simulink model "CryoDetXray"  (R2016b)
settings: Solver=ode45  StartTime=0.0  StopTime=10e-5  MaxStep=Tclk/4  RelTol=1e-3
values from neighbouring files (symbols this model uses):
  Fclk = Fadc    (= 307200000)    [setupCryoFPGAxray.m]
  Tclk = 1/Fclk    (= 3.25520833333e-09)    [setupCryoFPGAxray.m]
undefined symbols (not defined in the file or in its folder): AXI4, Lite, lpf, Naxi, xlipgetpartsetting
libraries: xbsIndex_r4 x1091, CryoDetLib x68, simulink x4, hdlsllib x1
(part 7 of 8)

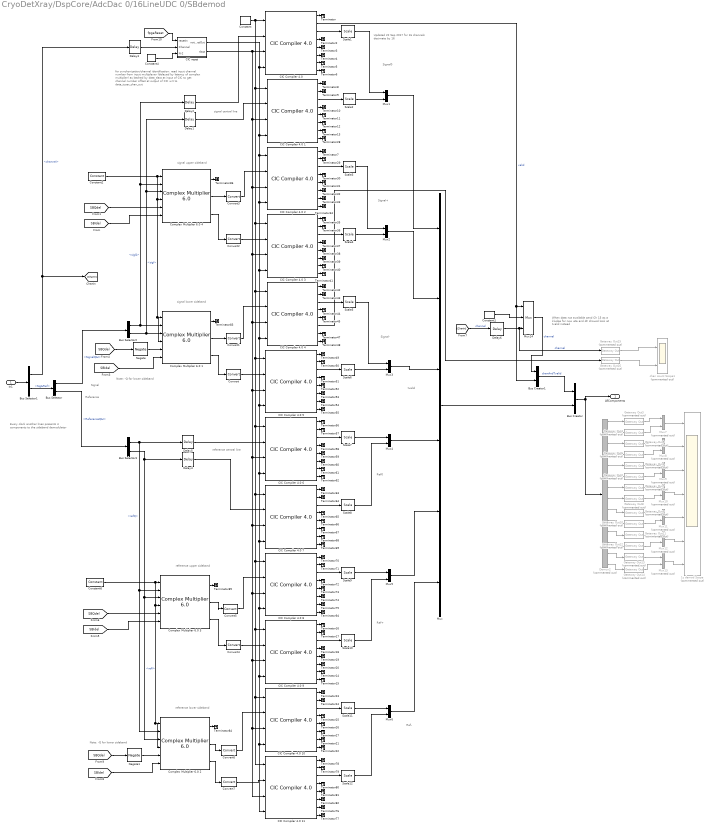
== system CryoDetXray/DspCore/AdcDac 0/16LineUDC 0/SBdemod ==
  note: Updated 22 Sep 2017 for 16 channels
      | decimate by 16
  note: When data not available send Ch 15 as
      | a kludge for now
      | eta and dF shouod look at tvalid instead
  note: tvalid
  note: Ref-
  note: Ref+
  note: Ref0
  note: Signal-
  note: Signal+
  note: Signal0
  note: for synchonization/channel identification:
      | read input channel number  from input multiplexer (delayed by latency of complex multiplier)
      | as latched by data_tlast at input of CIC to get channel number offset at output of CIC wrt to data_tuser_chan_out
  note: Note: -Q for lower sideband
  note: Every clock another lines presents 4 components to the sideband demodulator
  note: signal
      | central line
  note: signal
      | upper sideband
  note: signal
      | lower sideband
  note: Signal
  note: Reference
  note: reference
      | central line
  note: reference
      | upper sideband
  note: reference
      | lower sideband
  note: Note: -Q for lower sideband
  In1 : Inport
  1c demod Scope : Scope  Commented=on  NumInputPorts=7
  Bus Creator : BusCreator  Inputs=2
  Bus Creator1 : BusCreator  Inputs=2
  Bus Selector : BusSelector  OutputSignals=SignalQ&I,ReferenceQ&I
  Bus Selector1 : BusSelector  OutputSignals=channel,Sig&Ref
  Bus Selector2 : BusSelector  OutputSignals=sigQ,sigI
  Bus Selector3 : BusSelector  OutputSignals=refQ,refI
  CIC Compiler 4.0 {,1..11} (12 alike) : xbsIndex_r4/CIC Compiler 4.0   filter_type=Decimation  number_of_stages=3  differential_delay=1  number_of_channels=16  sample_rate_changes=Fixed  fixed_or_initial_rate=16  minimum_rate=16  maximum_rate=16  ratespecification=Sample_Period  sampleperiod=1  hardwareoversamplingrate=1  quantization=Truncation  output_data_width=24  use_xtreme_dsp_slice=off  use_streaming_interface=off  has_aclken=off  has_aresetn=on  has_dout_tready=off  trim_axipin_name=on  gui_behaviour=Sysgen_GUI  input_data_width=18  ip_name=CIC Compiler  ip_version=4.0  dsptool_ready=true  wrapper_available=true  port_translation_map={ 'aclken' => 'en', 'aresetn' => 'rst' }  ipcore_xco_need_fpga_part=true  ipcore_verbose=false  block_type=cic_compiler_v4_0
  CIC reset : Subsystem
  Complex Multiplier 6.0 {1..4} (4 alike) : xbsIndex_r4/Complex Multiplier 6.0   hasatlast=off  hasatuser=off  atuserwidth=1  hasbtlast=off  hasbtuser=off  btuserwidth=1  multtype=Use_Mults  optimizegoal=Resources  flowcontrol=NonBlocking  outputwidth=23  roundmode=Truncate  hasctrltlast=off  hasctrltuser=off  ctrltuserwidth=1  outtlastbehv=Null  latencyconfig=Manual  minimumlatency=6  aclken=off  aresetn=off  trim_axipin_name=on  simulation_type=hybrid_sim  simulation_model=sysgen:cmpy_v6_0  data_path_portlist={ 's_axis_a_tdata_real', 's_axis_a_tdata_imag', 's_axis_b_tdata_real', 's_axis_b_tdata_imag', 's_axis_ctrl_tdata_rounding_bit', 'm_axis_dout_tdata_real', 'm_axis_dout_tdata_imag' }  aportwidth=63  bportwidth=63  ip_name=Complex Multiplier  ip_version=6.0  dsptool_ready=true  ipcore_usecache=true  ipcore_useipmodelcache=true  ipcore_verbose=false  ipcore_latency_parameter='minimumlatency'  wrapper_available=true  port_translation_map={ 'aclken' => 'en', 'aresetn' => 'rst'}  block_type=cmpy_v6_0
  Constant : xbsIndex_r4/Constant  const=1.0  gui_display_data_type=Boolean  arith_type=Boolean  n_bits=16  bin_pt=14  preci_type=Single  exp_width=8  frac_width=24  explicit_period=off  period=1  equ=P=C  opselect=C  inp2=PCIN>>17  opr=+  inp1=P  carry=CIN  dbl_ovrd=off  block_type=constant
  Constant1 : xbsIndex_r4/Constant  const=15  gui_display_data_type=Fixed-point  arith_type=Unsigned  n_bits=4  bin_pt=0  preci_type=Single  exp_width=8  frac_width=24  explicit_period=off  period=1  equ=P=C  opselect=C  inp2=PCIN>>17  opr=+  inp1=P  carry=CIN  dbl_ovrd=off  block_type=constant
  Constant2 : xbsIndex_r4/Constant  const=1.0  gui_display_data_type=Boolean  arith_type=Boolean  n_bits=16  bin_pt=14  preci_type=Single  exp_width=8  frac_width=24  explicit_period=off  period=1  equ=P=C  opselect=C  inp2=PCIN>>17  opr=+  inp1=P  carry=CIN  dbl_ovrd=off  block_type=constant
  Constant4 : xbsIndex_r4/Constant  const=14  gui_display_data_type=Fixed-point  arith_type=Unsigned  n_bits=4  bin_pt=0  preci_type=Single  exp_width=8  frac_width=24  explicit_period=off  period=1  equ=P=C  opselect=C  inp2=PCIN>>17  opr=+  inp1=P  carry=CIN  dbl_ovrd=off  block_type=constant
  Constant6 : xbsIndex_r4/Constant  const=1.0  gui_display_data_type=Boolean  arith_type=Boolean  n_bits=16  bin_pt=14  preci_type=Single  exp_width=8  frac_width=24  explicit_period=off  period=1  equ=P=C  opselect=C  inp2=PCIN>>17  opr=+  inp1=P  carry=CIN  dbl_ovrd=off  block_type=constant
  Convert{,1..7} (8 alike) : xbsIndex_r4/Convert  gui_display_data_type=Fixed-point  arith_type="Signed  (2's comp)"  n_bits=20  bin_pt=16  float_type=Single  exp_bits=8  fraction_bits=24  quantization="Round  (unbiased: +/- Inf)"  overflow=Saturate  en=off  latency=0  pipeline=off  dbl_ovrd=off  block_type=convert
  Delay{1..2,4..5} (4 alike) : xbsIndex_r4/Delay  rst=off  infoeditControl=Selection of Reset will increase slice count due to use of real FFs and instead of SRLs  en=off  latency=6  reg_retiming=off  dbl_ovrd=off  block_type=delay
  Delay3 : xbsIndex_r4/Delay  rst=off  infoeditControl=Selection of Reset will increase slice count due to use of real FFs and instead of SRLs  en=off  latency=6  reg_retiming=on  dbl_ovrd=off  block_type=delay
  Delay6 : xbsIndex_r4/Delay  rst=off  infoeditControl=Selection of Reset will increase slice count due to use of real FFs and instead of SRLs  en=off  latency=4  reg_retiming=off  dbl_ovrd=off  block_type=delay
  Demux2 : Demux  Commented=on  Outputs=14
  Gateway Out{1..16} (16 alike) : xbsIndex_r4/Gateway Out  Commented=on  inherit_from_input=off  hdl_port=off  rows=1  columns=1  UseAsDAC=off  DACChannel='1'  interface=None  automatic_assignment=on  address_offset=hex2dec('00')  intf_name=''  intf_description=''  timing_constraint=None  locs_specified=off  LOCs={}  io_standard={}  block_type=gatewayout
  Mux : Mux  Inputs=6
  Mux{1..6} (6 alike) : Mux  Inputs=2
  Mux{7..13} (7 alike) : Mux  Commented=on  Inputs=2
  Mux14 : xbsIndex_r4/Mux  inputs=2  en=off  latency=0  precision=Full  arith_type=Unsigned  n_bits=16  bin_pt=14  quantization=Truncate  overflow=Wrap  dbl_ovrd=off  block_type=mux
  Negate : xbsIndex_r4/Negate  precision=User Defined  arith_type="Signed  (2's comp)"  n_bits=16  bin_pt=14  quantization=Truncate  overflow=Wrap  en=off  latency=0  dbl_ovrd=off  block_type=negate
  Negate1 : xbsIndex_r4/Negate  precision=User Defined  arith_type="Signed  (2's comp)"  n_bits=16  bin_pt=14  quantization=Truncate  overflow=Wrap  en=off  latency=0  dbl_ovrd=off  block_type=negate
  Scale{1..12} (12 alike) : xbsIndex_r4/Scale  scale_factor=-12  dbl_ovrd=off  block_type=scale
  Terminator{,2..45,47..86,94} (86 alike) : Terminator
  chan count Scope1 : Scope  Commented=on  NumInputPorts=2
  AllComponents : Outport
  wires:
  "CIC Compiler 4.0 "/3 -> Scale1/1
  Bus Selector/1 -> Bus Selector2/1  "<SignalQ&I>"
  Bus Selector2/1 -> Delay2/1, Complex Multiplier 6.0 4/2, Complex Multiplier 6.0 1/2  "<sigQ>"
  Bus Selector2/2 -> Complex Multiplier 6.0 4/3, Delay1/1, Complex Multiplier 6.0 1/3  "<sigI>"
  Bus Selector/2 -> Bus Selector3/1  "<ReferenceQ&I>"
  [SBIdel] -> Complex Multiplier 6.0 4/6
  [SBQdel] -> Complex Multiplier 6.0 4/5
  CIC reset/2(tlast) -> CIC Compiler 4.0 1/3, CIC Compiler 4.0 2/3, CIC Compiler 4.0 3/3, CIC Compiler 4.0 4/3, CIC Compiler 4.0 5/3, CIC Compiler 4.0 6/3, CIC Compiler 4.0 7/3, CIC Compiler 4.0 8/3, CIC Compiler 4.0 9/3, CIC Compiler 4.0 11/3, CIC Compiler 4.0 10/3, "CIC Compiler 4.0 "/3
  CIC reset/1(notResetOut) -> CIC Compiler 4.0 1/4, CIC Compiler 4.0 2/1, CIC Compiler 4.0 2/4, CIC Compiler 4.0 3/4, CIC Compiler 4.0 4/4, CIC Compiler 4.0 5/4, CIC Compiler 4.0 6/4, CIC Compiler 4.0 7/4, CIC Compiler 4.0 8/4, CIC Compiler 4.0 9/4, CIC Compiler 4.0 11/4, CIC Compiler 4.0 10/4, "CIC Compiler 4.0 "/4
  In1/1 -> Bus Selector1/1
  Bus Selector1/2 -> Bus Selector/1  "<Sig&Ref>"
  Delay1/1 -> CIC Compiler 4.0 1/2
  Delay2/1 -> "CIC Compiler 4.0 "/2
  Complex Multiplier 6.0 4/2 -> Convert3/1
  Complex Multiplier 6.0 4/3 -> Convert2/1
  Complex Multiplier 6.0 1/2 -> Convert1/1
  Complex Multiplier 6.0 1/3 -> Convert/1
  Constant2/1 -> Complex Multiplier 6.0 4/4, Complex Multiplier 6.0 1/4, Complex Multiplier 6.0 1/1, Complex Multiplier 6.0 4/1
  Bus Selector3/1 -> Complex Multiplier 6.0 2/2, Complex Multiplier 6.0 3/2, Delay5/1  "<refQ>"
  Bus Selector3/2 -> Complex Multiplier 6.0 2/3, Complex Multiplier 6.0 3/3, Delay4/1  "<refI>"
  [SBIdel] -> Complex Multiplier 6.0 3/6
  [SBQdel] -> Complex Multiplier 6.0 3/5
  Constant/1 -> "CIC Compiler 4.0 "/1, CIC Compiler 4.0 1/1, CIC Compiler 4.0 3/1, CIC Compiler 4.0 4/1, CIC Compiler 4.0 5/1, CIC Compiler 4.0 6/1, CIC Compiler 4.0 7/1, CIC Compiler 4.0 8/1, CIC Compiler 4.0 9/1, CIC Compiler 4.0 11/1, CIC Compiler 4.0 10/1
  Delay4/1 -> CIC Compiler 4.0 7/2
  Delay5/1 -> CIC Compiler 4.0 6/2
  Complex Multiplier 6.0 3/2 -> Convert5/1
  Complex Multiplier 6.0 3/3 -> Convert4/1
  Complex Multiplier 6.0 2/2 -> Convert6/1
  Complex Multiplier 6.0 2/3 -> Convert7/1
  Constant6/1 -> Complex Multiplier 6.0 3/4, Complex Multiplier 6.0 2/4, Complex Multiplier 6.0 2/1, Complex Multiplier 6.0 3/1
  Bus Selector1/1 -> Delay3/1, [ChanIn]  "<channel>"
  Delay3/1 -> CIC reset/2(Channel)
  Scale1/1 -> Mux1/1
  Scale6/1 -> Mux3/2
  Scale7/1 -> Mux4/1
  Scale8/1 -> Mux4/2
  Scale9/1 -> Mux5/1
  Scale10/1 -> Mux5/2
  Scale11/1 -> Mux6/1
  Scale12/1 -> Mux6/2
  Mux6/1 -> Mux/6
  Mux5/1 -> Mux/5
  Mux4/1 -> Mux/4
  Mux3/1 -> Mux/3
  Mux2/1 -> Mux/2
  Mux1/1 -> Mux/1
  Mux/1 -> Bus Creator/2
  [ChanIn] -> Delay6/1  "channel"
  Bus Creator1/1 -> Bus Creator/1  "chanAndTvalid"
  Convert/1 -> CIC Compiler 4.0 5/2
  Convert1/1 -> CIC Compiler 4.0 4/2
  Convert2/1 -> CIC Compiler 4.0 3/2
  Convert3/1 -> CIC Compiler 4.0 2/2
  Convert4/1 -> CIC Compiler 4.0 9/2
  Convert5/1 -> CIC Compiler 4.0 8/2
  Convert7/1 -> CIC Compiler 4.0 11/2
  Convert6/1 -> CIC Compiler 4.0 10/2
  Bus Creator/1 -> AllComponents/1, Demux2/1
  Demux2/1 -> Gateway Out3/1
  Demux2/2 -> Gateway Out4/1
  Demux2/3 -> Gateway Out5/1
  Demux2/4 -> Gateway Out6/1
  Gateway Out6/1 -> Mux8/2
  Gateway Out5/1 -> Mux8/1
  Gateway Out4/1 -> Mux7/2
  Gateway Out3/1 -> Mux7/1
  Mux7/1 -> 1c demod Scope/1
  Mux8/1 -> 1c demod Scope/2
  Demux2/14 -> Gateway Out14/1
  Demux2/13 -> Gateway Out13/1
  Gateway Out13/1 -> Mux13/1
  Gateway Out14/1 -> Mux13/2
  Mux13/1 -> 1c demod Scope/7
  Demux2/12 -> Gateway Out12/1
  Demux2/11 -> Gateway Out11/1
  Gateway Out11/1 -> Mux12/1
  Gateway Out12/1 -> Mux12/2
  Mux12/1 -> 1c demod Scope/6
  Demux2/10 -> Gateway Out10/1
  Demux2/9 -> Gateway Out9/1
  Gateway Out9/1 -> Mux11/1
  Gateway Out10/1 -> Mux11/2
  Mux11/1 -> 1c demod Scope/5
  Demux2/8 -> Gateway Out8/1
  Gateway Out8/1 -> Mux10/2
  Mux10/1 -> 1c demod Scope/4
  Gateway Out7/1 -> Mux10/1
  Demux2/7 -> Gateway Out7/1
  Demux2/6 -> Gateway Out2/1
  Gateway Out2/1 -> Mux9/2
  Gateway Out1/1 -> Mux9/1
  Demux2/5 -> Gateway Out1/1
  Mux9/1 -> 1c demod Scope/3
  Constant4/1 -> CIC reset/3(N-2)
  [fpgaReset] -> CIC reset/1(resetIn)
  Delay6/1 -> Gateway Out15/1, Mux14/3  "channel"
  Constant1/1 -> Mux14/2
  Mux14/1 -> Bus Creator1/1  "channel"
  [SBIdel] -> Complex Multiplier 6.0 1/6
  Negate/1 -> Complex Multiplier 6.0 1/5
  [SBQdel] -> Negate/1
  [SBIdel] -> Complex Multiplier 6.0 2/6
  [SBQdel] -> Negate1/1
  Negate1/1 -> Complex Multiplier 6.0 2/5
  "CIC Compiler 4.0 "/1 -> Terminator/1
  "CIC Compiler 4.0 "/2 -> Mux14/1, Bus Creator1/2  "valid"
  "CIC Compiler 4.0 "/4 -> Terminator2/1
  "CIC Compiler 4.0 "/5 -> Terminator3/1
  "CIC Compiler 4.0 "/6 -> Terminator4/1
  "CIC Compiler 4.0 "/7 -> Terminator5/1
  "CIC Compiler 4.0 "/8 -> Terminator6/1
  Complex Multiplier 6.0 1/1 -> Terminator83/1
  Complex Multiplier 6.0 2/1 -> Terminator84/1
  Complex Multiplier 6.0 3/1 -> Terminator85/1
  Complex Multiplier 6.0 4/1 -> Terminator86/1
  CIC Compiler 4.0 1/3 -> Scale2/1
  CIC Compiler 4.0 1/1 -> Terminator8/1
  CIC Compiler 4.0 1/2 -> Terminator9/1
  CIC Compiler 4.0 1/4 -> Terminator10/1
  CIC Compiler 4.0 1/5 -> Terminator11/1
  CIC Compiler 4.0 1/6 -> Terminator12/1
  CIC Compiler 4.0 1/7 -> Terminator13/1
  CIC Compiler 4.0 1/8 -> Terminator28/1
  CIC Compiler 4.0 2/3 -> Scale3/1
  CIC Compiler 4.0 2/1 -> Terminator7/1
  CIC Compiler 4.0 2/2 -> Terminator29/1
  CIC Compiler 4.0 2/4 -> Terminator30/1
  CIC Compiler 4.0 2/5 -> Terminator31/1
  CIC Compiler 4.0 2/6 -> Terminator32/1
  CIC Compiler 4.0 2/7 -> Terminator33/1
  CIC Compiler 4.0 2/8 -> Terminator34/1
  CIC Compiler 4.0 3/3 -> Scale4/1
  CIC Compiler 4.0 3/1 -> Terminator35/1
  CIC Compiler 4.0 3/2 -> Terminator36/1
  CIC Compiler 4.0 3/4 -> Terminator37/1
  CIC Compiler 4.0 3/5 -> Terminator38/1
  CIC Compiler 4.0 3/6 -> Terminator39/1
  CIC Compiler 4.0 3/7 -> Terminator40/1
  CIC Compiler 4.0 3/8 -> Terminator41/1
  CIC Compiler 4.0 4/3 -> Scale5/1
  CIC Compiler 4.0 4/1 -> Terminator42/1
  CIC Compiler 4.0 4/2 -> Terminator43/1
  CIC Compiler 4.0 4/4 -> Terminator44/1
  CIC Compiler 4.0 4/5 -> Terminator45/1
  CIC Compiler 4.0 4/7 -> Terminator47/1
  CIC Compiler 4.0 4/8 -> Terminator48/1
  Scale2/1 -> Mux1/2
  Scale3/1 -> Mux2/1
  Scale4/1 -> Mux2/2
  Scale5/1 -> Mux3/1
  CIC Compiler 4.0 5/3 -> Scale6/1
  CIC Compiler 4.0 5/1 -> Terminator49/1
  CIC Compiler 4.0 5/2 -> Terminator50/1
  CIC Compiler 4.0 5/4 -> Terminator51/1
  CIC Compiler 4.0 5/5 -> Terminator52/1
  CIC Compiler 4.0 5/6 -> Terminator53/1
  CIC Compiler 4.0 5/7 -> Terminator54/1
  CIC Compiler 4.0 5/8 -> Terminator55/1
  CIC Compiler 4.0 6/3 -> Scale7/1
  CIC Compiler 4.0 6/1 -> Terminator56/1
  CIC Compiler 4.0 6/2 -> Terminator57/1
  CIC Compiler 4.0 6/4 -> Terminator58/1
  CIC Compiler 4.0 6/5 -> Terminator59/1
  CIC Compiler 4.0 6/6 -> Terminator60/1
  CIC Compiler 4.0 6/7 -> Terminator61/1
  CIC Compiler 4.0 6/8 -> Terminator62/1
  CIC Compiler 4.0 7/3 -> Scale8/1
  CIC Compiler 4.0 7/1 -> Terminator63/1
  CIC Compiler 4.0 7/2 -> Terminator64/1
  CIC Compiler 4.0 7/4 -> Terminator65/1
  CIC Compiler 4.0 7/5 -> Terminator66/1
  CIC Compiler 4.0 7/6 -> Terminator67/1
  CIC Compiler 4.0 7/7 -> Terminator68/1
  CIC Compiler 4.0 7/8 -> Terminator69/1
  CIC Compiler 4.0 8/3 -> Scale9/1
  CIC Compiler 4.0 8/1 -> Terminator70/1
  CIC Compiler 4.0 8/2 -> Terminator71/1
  CIC Compiler 4.0 8/4 -> Terminator72/1
  CIC Compiler 4.0 8/5 -> Terminator73/1
  CIC Compiler 4.0 8/6 -> Terminator74/1
  CIC Compiler 4.0 8/7 -> Terminator75/1
  CIC Compiler 4.0 8/8 -> Terminator94/1
  CIC Compiler 4.0 9/3 -> Scale10/1
  CIC Compiler 4.0 9/1 -> Terminator16/1
  CIC Compiler 4.0 9/2 -> Terminator17/1
  CIC Compiler 4.0 9/4 -> Terminator18/1
  CIC Compiler 4.0 9/5 -> Terminator19/1
  CIC Compiler 4.0 9/6 -> Terminator20/1
  CIC Compiler 4.0 9/7 -> Terminator14/1
  CIC Compiler 4.0 9/8 -> Terminator15/1
  CIC Compiler 4.0 10/3 -> Scale11/1
  CIC Compiler 4.0 10/1 -> Terminator23/1
  CIC Compiler 4.0 10/2 -> Terminator24/1
  CIC Compiler 4.0 10/4 -> Terminator25/1
  CIC Compiler 4.0 10/5 -> Terminator26/1
  CIC Compiler 4.0 10/6 -> Terminator27/1
  CIC Compiler 4.0 10/7 -> Terminator21/1
  CIC Compiler 4.0 10/8 -> Terminator22/1
  CIC Compiler 4.0 11/3 -> Scale12/1
  CIC Compiler 4.0 11/1 -> Terminator78/1
  CIC Compiler 4.0 11/2 -> Terminator79/1
  CIC Compiler 4.0 11/4 -> Terminator80/1
  CIC Compiler 4.0 11/5 -> Terminator81/1
  CIC Compiler 4.0 11/6 -> Terminator82/1
  CIC Compiler 4.0 11/7 -> Terminator76/1
  CIC Compiler 4.0 11/8 -> Terminator77/1
  CIC Compiler 4.0 4/6 -> Gateway Out16/1
  Gateway Out15/1 -> chan count Scope1/1
  Gateway Out16/1 -> chan count Scope1/2

== system CryoDetXray/DspCore/AdcDac 0/16LineUDC 0/debug Scope ==
  note: Debug Demodulation
  demod : Inport
  freq : Inport  Port=2
  Complex to Magnitude-Angle : ComplexToMagnitudeAngle  Output=Magnitude
  Demux1 : Demux
  Gain : Gain  Gain=Fclk
  Gateway Out{1,3..6} (5 alike) : xbsIndex_r4/Gateway Out  inherit_from_input=off  hdl_port=off  rows=1  columns=1  UseAsDAC=off  DACChannel='1'  interface=None  automatic_assignment=on  address_offset=hex2dec('00')  intf_name=''  intf_description=''  timing_constraint=None  locs_specified=off  LOCs={}  io_standard={}  block_type=gatewayout
  Mux4 : Mux  Inputs=3
  Mux5 : Mux  Inputs=2
  Real-Imag to Complex : RealImagToComplex
  block downconverter Scope : Scope  NumInputPorts=3
  tag scope: FreqCh0=global
  wires:
  Gain/1 -> [FreqCh0], block downconverter Scope/3
  Gateway Out1/1 -> Gain/1
  freq/1 -> Gateway Out1/1
  Real-Imag to Complex/1 -> Complex to Magnitude-Angle/1
  Complex to Magnitude-Angle/1 -> Mux4/3
  Mux5/1 -> block downconverter Scope/2
  Mux4/1 -> block downconverter Scope/1
  Gateway Out3/1 -> Real-Imag to Complex/2, Mux4/1
  Gateway Out4/1 -> Real-Imag to Complex/1, Mux4/2
  Gateway Out5/1 -> Mux5/1
  Gateway Out6/1 -> Mux5/2
  Demux1/4 -> Gateway Out6/1
  Demux1/3 -> Gateway Out5/1
  Demux1/2 -> Gateway Out4/1
  Demux1/1 -> Gateway Out3/1
  demod/1 -> Demux1/1

== system CryoDetXray/DspCore/AdcDac 0/16ch LBW LPF/CIC reset ==
  note: where N is number of channels in CIC filter
  note: reset latched resetIn
  note: latch resetIn
  note: CIC reset
      |
      | Synchronizes a CIC compiler 4.0 multi-channel CIC filter
      | to input channels
      |
      | Generates:
      | 1	notResetOut to CIC aresetn
      | 2	tlast to CIC tlast input
      |
      | Inputs:
      | 1	reset in
      | 2	Channel number (0-N) which may go to sel input of mux generating the input data stream
      | 3	N-2 which tells this module how deep is the multiplexing (e.g. N-2 = 10 for a 12 channel CIC filter (sorry))
      |
      | Guarantees:
      | 1	reset out is at least 2 clocks long
      | 2	end of reset occurs 2 clocks before channel 0
      | 3	tlast comes with channel N-1
      |
      | Assumes:
      | CIC oversampling set to "Sample period" = 1
      | No "streaming interface"
  resetIn : Inport
  Channel : Inport  Port=2
  N-2 : Inport  Port=3
  Constant : xbsIndex_r4/Constant  const=0  gui_display_data_type=Boolean  arith_type=Boolean  n_bits=16  bin_pt=14  preci_type=Single  exp_width=8  frac_width=24  explicit_period=off  period=1  equ=P=C  opselect=C  inp2=PCIN>>17  opr=+  inp1=P  carry=CIN  dbl_ovrd=off  block_type=constant
  Delay1 : xbsIndex_r4/Delay  rst=off  infoeditControl=Selection of Reset will increase slice count due to use of real FFs and instead of SRLs  en=off  latency=1  reg_retiming=off  dbl_ovrd=off  block_type=delay
  Delay2 : xbsIndex_r4/Delay  rst=off  infoeditControl=Selection of Reset will increase slice count due to use of real FFs and instead of SRLs  en=off  latency=1  reg_retiming=off  dbl_ovrd=off  block_type=delay
  Delay3 : xbsIndex_r4/Delay  rst=off  infoeditControl=Selection of Reset will increase slice count due to use of real FFs and instead of SRLs  en=off  latency=1  reg_retiming=off  dbl_ovrd=off  block_type=delay
  Inverter : xbsIndex_r4/Inverter  en=off  latency=2  dbl_ovrd=off  block_type=inv
  Inverter1 : xbsIndex_r4/Inverter  en=off  latency=0  dbl_ovrd=off  block_type=inv
  Logical : xbsIndex_r4/Logical  logical_function=AND  inputs=4  en=off  latency=0  precision=User Defined  arith_type=Boolean  n_bits=1  bin_pt=0  align_bp=on  dbl_ovrd=off  block_type=logical
  Logical1 : xbsIndex_r4/Logical  logical_function=OR  inputs=2  en=off  latency=0  precision=User Defined  arith_type=Boolean  n_bits=1  bin_pt=0  align_bp=on  dbl_ovrd=off  block_type=logical
  Mux : xbsIndex_r4/Mux  inputs=2  en=off  latency=0  precision=Full  arith_type=Unsigned  n_bits=16  bin_pt=14  quantization=Truncate  overflow=Wrap  dbl_ovrd=off  block_type=mux
  Relational1 : xbsIndex_r4/Relational  mode=a=b  op_type=Bool  en=off  latency=0  dbl_ovrd=off  block_type=relational
  notResetOut : Outport
  tlast : Outport  Port=2
  wires:
  resetIn/1 -> Inverter/1, Logical1/1
  Channel/1 -> Relational1/1
  N-2/1 -> Relational1/2
  Relational1/1 -> Logical/4, Delay1/1
  Logical1/1 -> Inverter1/1, Delay2/1
  Mux/1 -> Logical1/2
  Delay2/1 -> Logical/2, Delay3/1, Mux/2
  Constant/1 -> Mux/3
  Logical/1 -> Mux/1
  Delay1/1 -> tlast/1
  Inverter/1 -> Logical/1
  Delay3/1 -> Logical/3
  Inverter1/1 -> notResetOut/1

== system CryoDetXray/DspCore/AdcDac 0/Flux Ramp DDC /CIC reset1 ==
  note: reset latch
  note: latch reset
  note: CIC reset
      |
      | Synchronizes a CIC compiler 4.0 multi-channel CIC filter
      | to input channels
      |
      | Generates:
      | notResetOut to CIC aresetn
      | talst to CIC talst input
      |
      | Inputs:
      | Channel number (0-N) which may go to sel input of mux generating the input data stream
      | N-2 which tells this module how deep is the multiplexing (e.g. N-2 = 10 for a 12 channel CIC filter (sorry))
      |
      | Guarantees:
      | 1	reset out is at least 2 clocks long
      | 2	end of reset occurs 2 clocks before channel 0
      | 3	tlast comes with channel N-1
      |
      | Assumes:
      | CIC oversampling set to "Sample period" = 1
      | No "streaming interface"
  resetIn : Inport
  Channel : Inport  Port=2
  N-2 : Inport  Port=3
  Constant : xbsIndex_r4/Constant  const=0  gui_display_data_type=Boolean  arith_type=Boolean  n_bits=16  bin_pt=14  preci_type=Single  exp_width=8  frac_width=24  explicit_period=off  period=1  equ=P=C  opselect=C  inp2=PCIN>>17  opr=+  inp1=P  carry=CIN  dbl_ovrd=off  block_type=constant
  Delay1 : xbsIndex_r4/Delay  rst=off  infoeditControl=Selection of Reset will increase slice count due to use of real FFs and instead of SRLs  en=off  latency=1  reg_retiming=off  dbl_ovrd=off  block_type=delay
  Delay2 : xbsIndex_r4/Delay  rst=off  infoeditControl=Selection of Reset will increase slice count due to use of real FFs and instead of SRLs  en=off  latency=1  reg_retiming=off  dbl_ovrd=off  block_type=delay
  Delay3 : xbsIndex_r4/Delay  rst=off  infoeditControl=Selection of Reset will increase slice count due to use of real FFs and instead of SRLs  en=off  latency=1  reg_retiming=off  dbl_ovrd=off  block_type=delay
  Inverter : xbsIndex_r4/Inverter  en=off  latency=2  dbl_ovrd=off  block_type=inv
  Inverter1 : xbsIndex_r4/Inverter  en=off  latency=0  dbl_ovrd=off  block_type=inv
  Logical : xbsIndex_r4/Logical  logical_function=AND  inputs=4  en=off  latency=0  precision=User Defined  arith_type=Boolean  n_bits=1  bin_pt=0  align_bp=on  dbl_ovrd=off  block_type=logical
  Logical1 : xbsIndex_r4/Logical  logical_function=OR  inputs=2  en=off  latency=0  precision=User Defined  arith_type=Boolean  n_bits=1  bin_pt=0  align_bp=on  dbl_ovrd=off  block_type=logical
  Mux : xbsIndex_r4/Mux  inputs=2  en=off  latency=0  precision=Full  arith_type=Unsigned  n_bits=16  bin_pt=14  quantization=Truncate  overflow=Wrap  dbl_ovrd=off  block_type=mux
  Relational1 : xbsIndex_r4/Relational  mode=a=b  op_type=Bool  en=off  latency=0  dbl_ovrd=off  block_type=relational
  notResetOut : Outport
  tlast : Outport  Port=2
  wires:
  resetIn/1 -> Inverter/1, Logical1/1
  Channel/1 -> Relational1/1
  N-2/1 -> Relational1/2
  Relational1/1 -> Logical/4, Delay1/1
  Logical1/1 -> Inverter1/1, Delay2/1
  Mux/1 -> Logical1/2
  Delay2/1 -> Logical/2, Delay3/1, Mux/2
  Constant/1 -> Mux/3
  Logical/1 -> Mux/1
  Delay1/1 -> tlast/1
  Inverter/1 -> Logical/1
  Delay3/1 -> Logical/3
  Inverter1/1 -> notResetOut/1

== system CryoDetXray/DspCore/AdcDac 0/FluxRamp/FM Amplitudes ==
  In1 : Inport
  Mux4 : xbsIndex_r4/Mux  inputs=16  en=off  latency=0  precision=Full  arith_type=Unsigned  n_bits=16  bin_pt=14  quantization=Truncate  overflow=Wrap  dbl_ovrd=off  block_type=mux
  Out1 : Outport
  wires:
  In1/1 -> Mux4/1
  Mux4/1 -> Out1/1
  [AFM4] -> Mux4/6
  [AFM1] -> Mux4/3
  [AFM8] -> Mux4/10
  [AFM3] -> Mux4/5
  [AFM0] -> Mux4/2
  [AFM2] -> Mux4/4
  [AFM9] -> Mux4/11
  [AFM7] -> Mux4/9
  [AFM11] -> Mux4/13
  [AFM6] -> Mux4/8
  [AFM5] -> Mux4/7
  [AFM10] -> Mux4/12
  [AFM13] -> Mux4/15
  [AFM14] -> Mux4/16
  [AFM15] -> Mux4/17
  [AFM12] -> Mux4/14

== system CryoDetXray/DspCore/AdcDac 0/FluxRamp/Flux Ramp Frequencies ==
  In1 : Inport
  Mux1 : xbsIndex_r4/Mux  inputs=16  en=off  latency=1  precision=Full  arith_type=Unsigned  n_bits=16  bin_pt=14  quantization=Truncate  overflow=Wrap  dbl_ovrd=off  block_type=mux
  Out1 : Outport
  wires:
  [wPhi9] -> Mux1/11
  [wPhi8] -> Mux1/10
  [wPhi7] -> Mux1/9
  [wPhi10] -> Mux1/12
  [wPhi11] -> Mux1/13
  [wPhi3] -> Mux1/5
  [wPhi0] -> Mux1/2
  [wPhi2] -> Mux1/4
  [wPhi1] -> Mux1/3
  Mux1/1 -> Out1/1
  [wPhi6] -> Mux1/8
  [wPhi5] -> Mux1/7
  [wPhi4] -> Mux1/6
  In1/1 -> Mux1/1
  [wPhi13] -> Mux1/15
  [wPhi12] -> Mux1/14
  [wPhi14] -> Mux1/16
  [wPhi15] -> Mux1/17

== system CryoDetXray/DspCore/AdcDac 0/FluxRamp/initial Frequencies ==
  note: initial Frequencies
  note: select initial frequency
      | for now just mux from input registers
      | eventually configure RAM and loading protocol
      | Now with latency 1
  channel : Inport
  BitBasher : xbsIndex_r4/BitBasher  bitexpr=a={b[24:24]}  display_expr=on  sr_1=a  arith_type1=Unsigned  bin_pt1=0  sr_2=2  arith_type2=Unsigned  bin_pt2=0  sr_3=3  arith_type3=Unsigned  bin_pt3=0  sr_4=4  arith_type4=Unsigned  bin_pt4=0  dbl_ovrd=off  block_type=bitbasher
  BitBasher1 : xbsIndex_r4/BitBasher  bitexpr=a={b[23:0]}  display_expr=on  sr_1=a  arith_type1=Unsigned  bin_pt1=24  sr_2=2  arith_type2=Unsigned  bin_pt2=0  sr_3=3  arith_type3=Unsigned  bin_pt3=0  sr_4=4  arith_type4=Unsigned  bin_pt4=0  dbl_ovrd=off  block_type=bitbasher
  Gateway Out12 : xbsIndex_r4/Gateway Out  inherit_from_input=off  hdl_port=off  rows=1  columns=1  UseAsDAC=off  DACChannel='1'  interface=None  automatic_assignment=on  address_offset=hex2dec('00')  intf_name=''  intf_description=''  timing_constraint=None  locs_specified=off  LOCs={}  io_standard={}  block_type=gatewayout
  Gateway Out13 : xbsIndex_r4/Gateway Out  inherit_from_input=off  hdl_port=off  rows=1  columns=1  UseAsDAC=off  DACChannel='1'  interface=None  automatic_assignment=on  address_offset=hex2dec('00')  intf_name=''  intf_description=''  timing_constraint=None  locs_specified=off  LOCs={}  io_standard={}  block_type=gatewayout
  Mux : xbsIndex_r4/Mux  inputs=16  en=off  latency=1  precision=Full  arith_type=Unsigned  n_bits=24  bin_pt=24  quantization=Truncate  overflow=Wrap  dbl_ovrd=off  block_type=mux
  initial Freqs : Scope  NumInputPorts=2
  Fi : Outport
  FBen : Outport  Port=2
  wires:
  channel/1 -> Gateway Out12/1, Mux/1
  [F0] -> Mux/2
  [F1] -> Mux/3
  [F2] -> Mux/4
  [F3] -> Mux/5
  [F4] -> Mux/6
  [F5] -> Mux/7
  [F6] -> Mux/8
  [F7] -> Mux/9
  [F8] -> Mux/10
  [F9] -> Mux/11
  [F10] -> Mux/12
  [F11] -> Mux/13
  Mux/1 -> BitBasher/1, BitBasher1/1
  Gateway Out13/1 -> initial Freqs/2
  Gateway Out12/1 -> initial Freqs/1
  BitBasher1/1 -> Gateway Out13/1, Fi/1
  BitBasher/1 -> FBen/1
  [F12] -> Mux/14
  [F13] -> Mux/15
  [F14] -> Mux/16
  [F15] -> Mux/17

== system CryoDetXray/DspCore/AdcDac 0/HBW Sig//Ref LPF/CIC reset ==
  note: where N is number of channels in CIC filter
  note: reset latched resetIn
  note: latch resetIn
  note: CIC reset
      |
      | Synchronizes a CIC compiler 4.0 multi-channel CIC filter
      | to input channels
      |
      | Generates:
      | 1	notResetOut to CIC aresetn
      | 2	tlast to CIC tlast input
      |
      | Inputs:
      | 1	reset in
      | 2	Channel number (0-N) which may go to sel input of mux generating the input data stream
      | 3	N-2 which tells this module how deep is the multiplexing (e.g. N-2 = 10 for a 12 channel CIC filter (sorry))
      |
      | Guarantees:
      | 1	reset out is at least 2 clocks long
      | 2	end of reset occurs 2 clocks before channel 0
      | 3	tlast comes with channel N-1
      |
      | Assumes:
      | CIC oversampling set to "Sample period" = 1
      | No "streaming interface"
  resetIn : Inport
  Channel : Inport  Port=2
  N-2 : Inport  Port=3
  Constant : xbsIndex_r4/Constant  const=0  gui_display_data_type=Boolean  arith_type=Boolean  n_bits=16  bin_pt=14  preci_type=Single  exp_width=8  frac_width=24  explicit_period=off  period=1  equ=P=C  opselect=C  inp2=PCIN>>17  opr=+  inp1=P  carry=CIN  dbl_ovrd=off  block_type=constant
  Delay1 : xbsIndex_r4/Delay  rst=off  infoeditControl=Selection of Reset will increase slice count due to use of real FFs and instead of SRLs  en=off  latency=1  reg_retiming=off  dbl_ovrd=off  block_type=delay
  Delay2 : xbsIndex_r4/Delay  rst=off  infoeditControl=Selection of Reset will increase slice count due to use of real FFs and instead of SRLs  en=off  latency=1  reg_retiming=off  dbl_ovrd=off  block_type=delay
  Delay3 : xbsIndex_r4/Delay  rst=off  infoeditControl=Selection of Reset will increase slice count due to use of real FFs and instead of SRLs  en=off  latency=1  reg_retiming=off  dbl_ovrd=off  block_type=delay
  Inverter : xbsIndex_r4/Inverter  en=off  latency=2  dbl_ovrd=off  block_type=inv
  Inverter1 : xbsIndex_r4/Inverter  en=off  latency=0  dbl_ovrd=off  block_type=inv
  Logical : xbsIndex_r4/Logical  logical_function=AND  inputs=4  en=off  latency=0  precision=User Defined  arith_type=Boolean  n_bits=1  bin_pt=0  align_bp=on  dbl_ovrd=off  block_type=logical
  Logical1 : xbsIndex_r4/Logical  logical_function=OR  inputs=2  en=off  latency=0  precision=User Defined  arith_type=Boolean  n_bits=1  bin_pt=0  align_bp=on  dbl_ovrd=off  block_type=logical
  Mux : xbsIndex_r4/Mux  inputs=2  en=off  latency=0  precision=Full  arith_type=Unsigned  n_bits=16  bin_pt=14  quantization=Truncate  overflow=Wrap  dbl_ovrd=off  block_type=mux
  Relational1 : xbsIndex_r4/Relational  mode=a=b  op_type=Bool  en=off  latency=0  dbl_ovrd=off  block_type=relational
  notResetOut : Outport
  tlast : Outport  Port=2
  wires:
  resetIn/1 -> Inverter/1, Logical1/1
  Channel/1 -> Relational1/1
  N-2/1 -> Relational1/2
  Relational1/1 -> Logical/4, Delay1/1
  Logical1/1 -> Inverter1/1, Delay2/1
  Mux/1 -> Logical1/2
  Delay2/1 -> Logical/2, Delay3/1, Mux/2
  Constant/1 -> Mux/3
  Logical/1 -> Mux/1
  Delay1/1 -> tlast/1
  Inverter/1 -> Logical/1
  Delay3/1 -> Logical/3
  Inverter1/1 -> notResetOut/1

== system CryoDetXray/DspCore/AdcDac 0/S21/Complex Divide ==
  note: Complex multiplier has latency 6
  a_tvalid : Inport
  A_Q : Inport  Port=2
  A_I : Inport  Port=3
  b_tvalid : Inport  Port=4
  B_Q : Inport  Port=5
  B_I : Inport  Port=6
  AddSub : xbsIndex_r4/AddSub  mode=Addition  use_carryin=off  use_carryout=off  en=off  latency=3  precision=Full  arith_type="Signed  (2's comp)"  n_bits=48  bin_pt=44  quantization=Truncate  overflow=Flag as error  use_behavioral_HDL=on  hw_selection=Fabric  pipelined=off  dbl_ovrd=off  block_type=addsub
  CMult : xbsIndex_r4/CMult  const=-1  gui_display_data_type=Floating-point  const_n_bits=16  const_bin_pt=15  float_type=Single  exp_bits=8  fraction_bits=24  en=off  latency=3  precision=Full  arith_type="Signed  (2's comp)"  n_bits=32  bin_pt=30  quantization=Truncate  overflow=Wrap  use_behavioral_HDL=off  mem_type=Distributed RAM  pipeline=off  dbl_ovrd=off  block_type=cmult
  Constant : xbsIndex_r4/Constant  const=0  gui_display_data_type=Floating-point  arith_type=Floating-point  n_bits=63  bin_pt=15  preci_type=Single  exp_width=8  frac_width=24  explicit_period=off  period=1  equ=P=C  opselect=C  inp2=PCIN>>17  opr=+  inp1=P  carry=CIN  dbl_ovrd=off  block_type=constant
  Cplx Div 2 : Scope  Commented=on  NumInputPorts=3
  CplxProd : Subsystem
  Cpx Div : Scope  Commented=on  NumInputPorts=4
  Delay{,1..2,5} (4 alike) : xbsIndex_r4/Delay  rst=off  infoeditControl=Selection of Reset will increase slice count due to use of real FFs and instead of SRLs  en=off  latency=3  reg_retiming=on  dbl_ovrd=off  block_type=delay
  Delay3 : xbsIndex_r4/Delay  rst=off  infoeditControl=Selection of Reset will increase slice count due to use of real FFs and instead of SRLs  en=off  latency=12  reg_retiming=on  dbl_ovrd=off  block_type=delay
  Delay{4,6..8} (4 alike) : xbsIndex_r4/Delay  rst=off  infoeditControl=Selection of Reset will increase slice count due to use of real FFs and instead of SRLs  en=off  latency=2  reg_retiming=on  dbl_ovrd=off  block_type=delay
  Delay9 : xbsIndex_r4/Delay  rst=off  infoeditControl=Selection of Reset will increase slice count due to use of real FFs and instead of SRLs  en=off  latency=1  reg_retiming=on  dbl_ovrd=off  block_type=delay
  Divide : xbsIndex_r4/Divide  flow_control=NonBlocking  axi_optimize_goal=Resources  algorithm_type=Radix2  infoedit1=Specify output fraction-width for Fixed-point division.  fractional_width=24  infoedit2=Specify latency for Floating-point division.  latency=12  rate=1  has_a_tlast=off  has_a_tuser=off  has_b_tlast=off  has_b_tuser=off  en=off  has_result_tready=off  result_tlast_behv=Pass_A_TLAST  has_underflow=on  has_overflow=on  has_invalid_op=on  has_divide_by_zero=on  fpo_op_type=mergeddivide  block_type=divide
      settings: infoedit=Blocking: Wait for data on all inputs, allow back-pressure.<br>NonBlocking: operate every cycle in which all inputs are valid, no back-pressure.
  Divide1 : xbsIndex_r4/Divide  flow_control=NonBlocking  axi_optimize_goal=Resources  algorithm_type=Radix2  infoedit1=Specify output fraction-width for Fixed-point division.  fractional_width=24  infoedit2=Specify latency for Floating-point division.  latency=12  rate=1  has_a_tlast=off  has_a_tuser=off  has_b_tlast=off  has_b_tuser=off  en=off  has_result_tready=off  result_tlast_behv=Pass_A_TLAST  has_underflow=on  has_overflow=on  has_invalid_op=on  has_divide_by_zero=on  fpo_op_type=mergeddivide  block_type=divide
      settings: infoedit=Blocking: Wait for data on all inputs, allow back-pressure.<br>NonBlocking: operate every cycle in which all inputs are valid, no back-pressure.
  Gateway Out{1..2,6..12,14..17} (13 alike) : xbsIndex_r4/Gateway Out  Commented=on  inherit_from_input=off  hdl_port=off  rows=1  columns=1  UseAsDAC=off  DACChannel='1'  interface=None  automatic_assignment=on  address_offset=hex2dec('00')  intf_name=''  intf_description=''  timing_constraint=None  locs_specified=off  LOCs={}  io_standard={}  block_type=gatewayout
  Mult : xbsIndex_r4/Mult  precision=Full  arith_type="Signed  (2's comp)"  n_bits=48  bin_pt=44  quantization=Truncate  overflow=Flag as error  en=off  latency=6  use_behavioral_HDL=on  opt=Speed  use_embedded=on  optimum_pipeline=on  pipeline=on  dbl_ovrd=off  use_rpm=on  placement_style=Triangular  block_type=mult
  Mult1 : xbsIndex_r4/Mult  precision=Full  arith_type="Signed  (2's comp)"  n_bits=48  bin_pt=44  quantization=Truncate  overflow=Flag as error  en=off  latency=6  use_behavioral_HDL=on  opt=Speed  use_embedded=on  optimum_pipeline=off  pipeline=on  dbl_ovrd=off  use_rpm=on  placement_style=Triangular  block_type=mult
  Mux{1,3..5,9..10} (6 alike) : Mux  Commented=on  Inputs=2
  Mux6 : xbsIndex_r4/Mux  inputs=2  en=off  latency=0  precision=Full  arith_type=Unsigned  n_bits=63  bin_pt=15  quantization=Truncate  overflow=Flag as error  dbl_ovrd=off  block_type=mux
  Mux7 : xbsIndex_r4/Mux  inputs=2  en=off  latency=1  precision=Full  arith_type=Unsigned  n_bits=63  bin_pt=15  quantization=Truncate  overflow=Flag as error  dbl_ovrd=off  block_type=mux
  Terminator{,1..3,5} (5 alike) : Terminator
  tvalidOut : Outport
  Out_Q : Outport  Port=2
  Out_I : Outport  Port=3
  invalid op : Outport  Port=4
  wires:
  a_tvalid/1 -> Gateway Out12/1, Delay/1
  A_Q/1 -> Delay1/1, Gateway Out14/1
  A_I/1 -> Delay2/1, Gateway Out15/1
  Divide/1 -> Mux7/2
  Mult1/1 -> AddSub/2
  AddSub/1 -> Delay8/1
  Divide1/4 -> Gateway Out11/1, invalid op/1, Mux6/1, Mux7/1
  Mux7/1 -> Gateway Out6/1, Out_Q/1
  Mux6/1 -> Out_I/1, Gateway Out7/1
  Mult/1 -> AddSub/1
  Gateway Out6/1 -> Mux3/1
  Gateway Out7/1 -> Mux3/2
  Gateway Out8/1 -> Mux4/1
  Gateway Out9/1 -> Mux4/2
  Gateway Out10/1 -> Mux5/1
  Gateway Out11/1 -> Mux5/2
  Divide1/1 -> Mux6/2
  Constant/1 -> Mux7/3, Mux6/3
  Delay5/1 -> CplxProd/5(Re_B)
  Delay2/1 -> CplxProd/3(Re_A)
  Delay1/1 -> CplxProd/2(Im_A)
  Delay/1 -> CplxProd/1(tvalidIn)
  B_Q/1 -> Mult1/1, Mult1/2, Gateway Out16/1, CMult/1
  B_I/1 -> Mult/1, Mult/2, Delay5/1, Gateway Out17/1
  CMult/1 -> CplxProd/4(Im_B)
  Gateway Out14/1 -> Mux9/1
  Gateway Out15/1 -> Mux9/2
  Gateway Out16/1 -> Mux10/1
  Gateway Out17/1 -> Mux10/2
  Gateway Out12/1 -> Cplx Div 2/1
  Mux9/1 -> Cplx Div 2/2
  Mux10/1 -> Cplx Div 2/3
  b_tvalid/1 -> Terminator5/1
  CplxProd/2(Im_Out) -> Delay6/1
  CplxProd/1(tvalidOut) -> Delay4/1
  CplxProd/3(Re_Out) -> Delay7/1
  Divide1/2 -> Gateway Out8/1
  Divide1/3 -> Gateway Out9/1
  Divide1/5 -> Gateway Out10/1
  Mux3/1 -> Cpx Div/2
  Mux4/1 -> Cpx Div/3
  Mux5/1 -> Cpx Div/4
  Delay3/1 -> Delay9/1
  Mux1/1 -> Cpx Div/1
  Divide/2 -> Terminator/1
  Divide/3 -> Terminator1/1
  Divide/4 -> Terminator2/1
  Divide/5 -> Terminator3/1
  Gateway Out2/1 -> Mux1/2
  Gateway Out1/1 -> Mux1/1
  Delay4/1 -> Gateway Out1/1, Delay3/1
  Delay6/1 -> Divide/1
  Delay7/1 -> Divide1/1
  Delay8/1 -> Divide/2, Divide1/2
  Delay9/1 -> Gateway Out2/1, tvalidOut/1

== system CryoDetXray/DspCore/AdcDac 0/S21/IIR LPF ==
  note: Reasonably valid data ?
  chanIn : Inport
  Qin : Inport  Port=2
  Iin : Inport  Port=3
  inavalidIn : Inport  Port=4
  Absolute : xbsIndex_r4/Absolute  precision=Full  arith_type=Unsigned  n_bits=16  bin_pt=14  quantization=Truncate  overflow=Wrap  en=off  latency=1  dbl_ovrd=off  block_type=abs
  Absolute1 : xbsIndex_r4/Absolute  precision=Full  arith_type=Unsigned  n_bits=16  bin_pt=14  quantization=Truncate  overflow=Wrap  en=off  latency=1  dbl_ovrd=off  block_type=abs
  AddSub : xbsIndex_r4/AddSub  mode=Addition  use_carryin=off  use_carryout=off  en=off  latency=4  precision=Full  arith_type="Signed  (2's comp)"  n_bits=24  bin_pt=16  quantization=Truncate  overflow=Saturate  use_behavioral_HDL=on  hw_selection=Fabric  pipelined=off  dbl_ovrd=off  block_type=addsub
  AddSub1 : xbsIndex_r4/AddSub  mode=Subtraction  use_carryin=off  use_carryout=off  en=off  latency=4  precision=Full  arith_type=Unsigned  n_bits=16  bin_pt=14  quantization=Truncate  overflow=Wrap  use_behavioral_HDL=on  hw_selection=Fabric  pipelined=off  dbl_ovrd=off  block_type=addsub
  AddSub2 : xbsIndex_r4/AddSub  mode=Addition  use_carryin=off  use_carryout=off  en=off  latency=4  precision=Full  arith_type="Signed  (2's comp)"  n_bits=24  bin_pt=16  quantization=Truncate  overflow=Saturate  use_behavioral_HDL=on  hw_selection=Fabric  pipelined=off  dbl_ovrd=off  block_type=addsub
  AddSub3 : xbsIndex_r4/AddSub  mode=Addition  use_carryin=off  use_carryout=off  en=off  latency=4  precision=Full  arith_type=Unsigned  n_bits=16  bin_pt=14  quantization=Truncate  overflow=Wrap  use_behavioral_HDL=off  hw_selection=Fabric  pipelined=off  dbl_ovrd=off  block_type=addsub
  Complex to Magnitude-Angle : ComplexToMagnitudeAngle
  Complex to Magnitude-Angle1 : ComplexToMagnitudeAngle
  Constant : xbsIndex_r4/Constant  const=1  gui_display_data_type=Floating-point  arith_type=Floating-point  n_bits=16  bin_pt=14  preci_type=Single  exp_width=8  frac_width=24  explicit_period=off  period=1  equ=P=C  opselect=C  inp2=PCIN>>17  opr=+  inp1=P  carry=CIN  dbl_ovrd=off  block_type=constant
  Constant1 : xbsIndex_r4/Constant  const=1e5  gui_display_data_type=Floating-point  arith_type=Floating-point  n_bits=16  bin_pt=14  preci_type=Single  exp_width=8  frac_width=24  explicit_period=off  period=1  equ=P=C  opselect=C  inp2=PCIN>>17  opr=+  inp1=P  carry=CIN  dbl_ovrd=off  block_type=constant
  Constant2 : xbsIndex_r4/Constant  const=0  gui_display_data_type=Floating-point  arith_type=Floating-point  n_bits=16  bin_pt=14  preci_type=Single  exp_width=8  frac_width=24  explicit_period=off  period=1  equ=P=C  opselect=C  inp2=PCIN>>17  opr=+  inp1=P  carry=CIN  dbl_ovrd=off  block_type=constant
  Constant3 : xbsIndex_r4/Constant  const=0  gui_display_data_type=Fixed-point  arith_type=Unsigned  n_bits=16  bin_pt=16  preci_type=Single  exp_width=8  frac_width=24  explicit_period=off  period=1  equ=P=C  opselect=C  inp2=PCIN>>17  opr=+  inp1=P  carry=CIN  dbl_ovrd=off  block_type=constant
  Constant4 : xbsIndex_r4/Constant  const=1  gui_display_data_type=Fixed-point  arith_type=Unsigned  n_bits=16  bin_pt=16  preci_type=Single  exp_width=8  frac_width=24  explicit_period=off  period=1  equ=P=C  opselect=C  inp2=PCIN>>17  opr=+  inp1=P  carry=CIN  dbl_ovrd=off  block_type=constant
  Constant5 : xbsIndex_r4/Constant  const=0  gui_display_data_type=Floating-point  arith_type=Floating-point  n_bits=16  bin_pt=14  preci_type=Single  exp_width=8  frac_width=24  explicit_period=off  period=1  equ=P=C  opselect=C  inp2=PCIN>>17  opr=+  inp1=P  carry=CIN  dbl_ovrd=off  block_type=constant
  Convert : xbsIndex_r4/Convert  gui_display_data_type=Floating-point  arith_type=Floating-point  n_bits=16  bin_pt=14  float_type=Single  exp_bits=8  fraction_bits=24  quantization=Truncate  overflow=Wrap  en=off  latency=2  pipeline=off  dbl_ovrd=off  block_type=convert
  Convert1 : xbsIndex_r4/Convert  gui_display_data_type=Fixed-point  arith_type="Signed  (2's comp)"  n_bits=18  bin_pt=16  float_type=Single  exp_bits=8  fraction_bits=24  quantization=Truncate  overflow=Wrap  en=off  latency=1  pipeline=off  dbl_ovrd=off  block_type=convert
  Delay : xbsIndex_r4/Delay  rst=off  infoeditControl=Selection of Reset will increase slice count due to use of real FFs and instead of SRLs  en=off  latency=3  reg_retiming=off  dbl_ovrd=off  block_type=delay
  Delay1 : xbsIndex_r4/Delay  rst=off  infoeditControl=Selection of Reset will increase slice count due to use of real FFs and instead of SRLs  en=off  latency=3  reg_retiming=off  dbl_ovrd=off  block_type=delay
  Delay2 : xbsIndex_r4/Delay  rst=off  infoeditControl=Selection of Reset will increase slice count due to use of real FFs and instead of SRLs  en=off  latency=8  reg_retiming=off  dbl_ovrd=off  block_type=delay
  Delay3 : xbsIndex_r4/Delay  rst=off  infoeditControl=Selection of Reset will increase slice count due to use of real FFs and instead of SRLs  en=off  latency=9  reg_retiming=on  dbl_ovrd=off  block_type=delay
  Delay4 : xbsIndex_r4/Delay  rst=off  infoeditControl=Selection of Reset will increase slice count due to use of real FFs and instead of SRLs  en=off  latency=9  reg_retiming=on  dbl_ovrd=off  block_type=delay
  Delay5 : xbsIndex_r4/Delay  rst=off  infoeditControl=Selection of Reset will increase slice count due to use of real FFs and instead of SRLs  en=off  latency=1  reg_retiming=off  dbl_ovrd=off  block_type=delay
  Display : Display
  Display1 : Display
  Gateway Out{,1..8} (9 alike) : xbsIndex_r4/Gateway Out  inherit_from_input=off  hdl_port=off  rows=1  columns=1  UseAsDAC=off  DACChannel='1'  interface=None  automatic_assignment=on  address_offset=hex2dec('00')  intf_name=''  intf_description=''  timing_constraint=None  locs_specified=off  LOCs={}  io_standard={}  block_type=gatewayout
  Logical : xbsIndex_r4/Logical  logical_function=AND  inputs=2  en=off  latency=1  precision=Full  arith_type=Unsigned  n_bits=16  bin_pt=0  align_bp=on  dbl_ovrd=off  block_type=logical
  Mult : xbsIndex_r4/Mult  precision=Full  arith_type="Signed  (2's comp)"  n_bits=16  bin_pt=14  quantization=Truncate  overflow=Wrap  en=off  latency=3  use_behavioral_HDL=off  opt=Speed  use_embedded=on  optimum_pipeline=off  pipeline=on  dbl_ovrd=off  use_rpm=on  placement_style=Triangular  block_type=mult
  Mult1 : xbsIndex_r4/Mult  precision=Full  arith_type="Signed  (2's comp)"  n_bits=16  bin_pt=14  quantization=Truncate  overflow=Wrap  en=off  latency="16*8 -  4 - 1"  use_behavioral_HDL=off  opt=Speed  use_embedded=on  optimum_pipeline=off  pipeline=on  dbl_ovrd=off  use_rpm=on  placement_style=Triangular  block_type=mult
  Mult2 : xbsIndex_r4/Mult  precision=Full  arith_type="Signed  (2's comp)"  n_bits=16  bin_pt=14  quantization=Truncate  overflow=Wrap  en=off  latency=3  use_behavioral_HDL=off  opt=Speed  use_embedded=on  optimum_pipeline=off  pipeline=on  dbl_ovrd=off  use_rpm=on  placement_style=Triangular  block_type=mult
  Mult3 : xbsIndex_r4/Mult  precision=Full  arith_type="Signed  (2's comp)"  n_bits=16  bin_pt=14  quantization=Truncate  overflow=Wrap  en=off  latency="16*8 -  4 - 1"  use_behavioral_HDL=off  opt=Speed  use_embedded=on  optimum_pipeline=off  pipeline=on  dbl_ovrd=off  use_rpm=on  placement_style=Triangular  block_type=mult
  Mux{,1..4} (5 alike) : xbsIndex_r4/Mux  inputs=2  en=off  latency=1  precision=Full  arith_type=Unsigned  n_bits=16  bin_pt=14  quantization=Truncate  overflow=Wrap  dbl_ovrd=off  block_type=mux
  Real-Imag to Complex : RealImagToComplex
  Real-Imag to Complex1 : RealImagToComplex
  Relational : xbsIndex_r4/Relational  mode=a<b  op_type=Bool  en=off  latency=3  dbl_ovrd=off  block_type=relational
  Relational1 : xbsIndex_r4/Relational  mode=a=b  op_type=Bool  en=off  latency=1  dbl_ovrd=off  block_type=relational
  S21 lpf Scope : Scope  NumInputPorts=4
  S21 lpf input qualifier : Scope  NumInputPorts=4
  mag S21 in : Display
  mag S21 out : Display
  chanOut : Outport
  Qout : Outport  Port=2
  Iout : Outport  Port=3
  wires:
  chanIn/1 -> Delay2/1
  Constant/1 -> AddSub1/1
  Convert/1 -> AddSub1/2, Gateway Out7/1, Mult2/1, Mult/1
  AddSub/1 -> Mux3/2, Mult/2
  Mult1/1 -> AddSub/2
  Qin/1 -> Absolute/1, Delay3/1
  AddSub1/1 -> Mult3/2, Mult1/2, Gateway Out8/1
  Mult/1 -> Gateway Out3/1, Qout/1
  Delay/1 -> Delay1/1
  Delay1/1 -> chanOut/1
  AddSub2/1 -> Mux4/2, Mult2/2
  Mult3/1 -> AddSub2/2
  Iin/1 -> Delay4/1, Absolute1/1
  Mult2/1 -> Gateway Out2/1, Iout/1
  Real-Imag to Complex/1 -> Complex to Magnitude-Angle/1
  Gateway Out1/1 -> Real-Imag to Complex/1
  Gateway Out/1 -> Real-Imag to Complex/2
  Real-Imag to Complex1/1 -> Complex to Magnitude-Angle1/1
  Gateway Out3/1 -> Real-Imag to Complex1/1
  Gateway Out2/1 -> Real-Imag to Complex1/2
  Complex to Magnitude-Angle/2 -> S21 lpf Scope/4
  Complex to Magnitude-Angle/1 -> S21 lpf input qualifier/1, mag S21 in/1, S21 lpf Scope/3
  Complex to Magnitude-Angle1/1 -> S21 lpf Scope/1, mag S21 out/1
  Complex to Magnitude-Angle1/2 -> S21 lpf Scope/2
  Convert1/1 -> Convert/1
  Absolute1/1 -> AddSub3/1
  Absolute/1 -> AddSub3/2
  Relational/1 -> Logical/2
  AddSub3/1 -> Relational/2
  Constant1/1 -> Relational/1
  inavalidIn/1 -> Logical/1
  Mux/1 -> AddSub/1, Gateway Out1/1
  Logical/1 -> Mux1/1, Mux/1, Gateway Out4/1
  Mux1/1 -> Gateway Out/1, AddSub2/1
  Constant2/1 -> Mux1/3, Mux/3
  Delay2/1 -> Delay5/1
  Delay3/1 -> Mux/2, Gateway Out6/1
  Delay4/1 -> Mux1/2, Gateway Out5/1
  Gateway Out4/1 -> S21 lpf input qualifier/4
  Gateway Out5/1 -> S21 lpf input qualifier/2
  Gateway Out6/1 -> S21 lpf input qualifier/3
  Gateway Out8/1 -> Display/1
  Gateway Out7/1 -> Display1/1
  Constant3/1 -> Relational1/1
  Relational1/1 -> Mux2/1
  Constant4/1 -> Mux2/3
  [omegaTsPhiRef] -> Relational1/2, Mux2/2
  Mux2/1 -> Convert1/1
  Mux4/1 -> Mult3/1
  Mux3/1 -> Mult1/1
  [FBreset] -> Mux4/1, Mux3/1
  Constant5/1 -> Mux4/3, Mux3/3
  Delay5/1 -> Delay/1

== system CryoDetXray/DspCore/AdcDac 0/dF1/eta Mux ==
  note: eta Mux
  note: get calibration const for this channel
      | for now just mux from input registers
      | eventually configure RAM and loading protocol
  channel : Inport
  Bus Creator : BusCreator  Inputs=2
  Gateway Out1 : xbsIndex_r4/Gateway Out  inherit_from_input=off  hdl_port=off  rows=1  columns=1  UseAsDAC=off  DACChannel='1'  interface=None  automatic_assignment=on  address_offset=hex2dec('00')  intf_name=''  intf_description=''  timing_constraint=None  locs_specified=off  LOCs={}  io_standard={}  block_type=gatewayout
  Gateway Out12 : xbsIndex_r4/Gateway Out  inherit_from_input=off  hdl_port=off  rows=1  columns=1  UseAsDAC=off  DACChannel='1'  interface=None  automatic_assignment=on  address_offset=hex2dec('00')  intf_name=''  intf_description=''  timing_constraint=None  locs_specified=off  LOCs={}  io_standard={}  block_type=gatewayout
  Gateway Out13 : xbsIndex_r4/Gateway Out  inherit_from_input=off  hdl_port=off  rows=1  columns=1  UseAsDAC=off  DACChannel='1'  interface=None  automatic_assignment=on  address_offset=hex2dec('00')  intf_name=''  intf_description=''  timing_constraint=None  locs_specified=off  LOCs={}  io_standard={}  block_type=gatewayout
  Mux : xbsIndex_r4/Mux  inputs=16  en=off  latency=1  precision=Full  arith_type=Unsigned  n_bits=24  bin_pt=24  quantization=Truncate  overflow=Wrap  dbl_ovrd=off  block_type=mux
  Mux1 : xbsIndex_r4/Mux  inputs=16  en=off  latency=1  precision=Full  arith_type=Unsigned  n_bits=24  bin_pt=24  quantization=Truncate  overflow=Wrap  dbl_ovrd=off  block_type=mux
  eta scope : Scope  NumInputPorts=3
  eta out : Outport
  wires:
  channel/1 -> Mux/1, Gateway Out12/1, Mux1/1
  [reEta0] -> Mux/2
  [reEta1] -> Mux/3
  [reEta2] -> Mux/4
  [reEta3] -> Mux/5
  [reEta4] -> Mux/6
  [reEta5] -> Mux/7
  [reEta6] -> Mux/8
  [reEta7] -> Mux/9
  [reEta8] -> Mux/10
  [reEta9] -> Mux/11
  [reEta10] -> Mux/12
  [reEta11] -> Mux/13
  Mux/1 -> Bus Creator/1, Gateway Out13/1  "reEta"
  Gateway Out13/1 -> eta scope/2
  Gateway Out12/1 -> eta scope/1
  [imEta0] -> Mux1/2
  [imEta1] -> Mux1/3
  [imEta2] -> Mux1/4
  [imEta3] -> Mux1/5
  [imEta4] -> Mux1/6
  [imEta5] -> Mux1/7
  [imEta6] -> Mux1/8
  [imEta7] -> Mux1/9
  [imEta8] -> Mux1/10
  [imEta9] -> Mux1/11
  [imEta10] -> Mux1/12
  [imEta11] -> Mux1/13
  Mux1/1 -> Bus Creator/2, Gateway Out1/1  "imEta"
  Gateway Out1/1 -> eta scope/3
  Bus Creator/1 -> eta out/1
  [reEta15] -> Mux/17
  [reEta14] -> Mux/16
  [reEta13] -> Mux/15
  [reEta12] -> Mux/14
  [imEta12] -> Mux1/14
  [imEta13] -> Mux1/15
  [imEta14] -> Mux1/16
  [imEta15] -> Mux1/17
